simulink model "comp_ctrl"  (R2020b)
settings: Solver=VariableStepAuto  StartTime=0.0  StopTime=2e-3  MaxStep=1e-5  RelTol=1e-3
undefined symbols (not defined in the file or in its folder): den_cos, den_d, L_d, num_cos, num_d, R_s, t_s
libraries: simulink x2
settings Model: PauseTimes=2e-3  Creator=LaptopBN  LastModifiedBy=LaptopBN

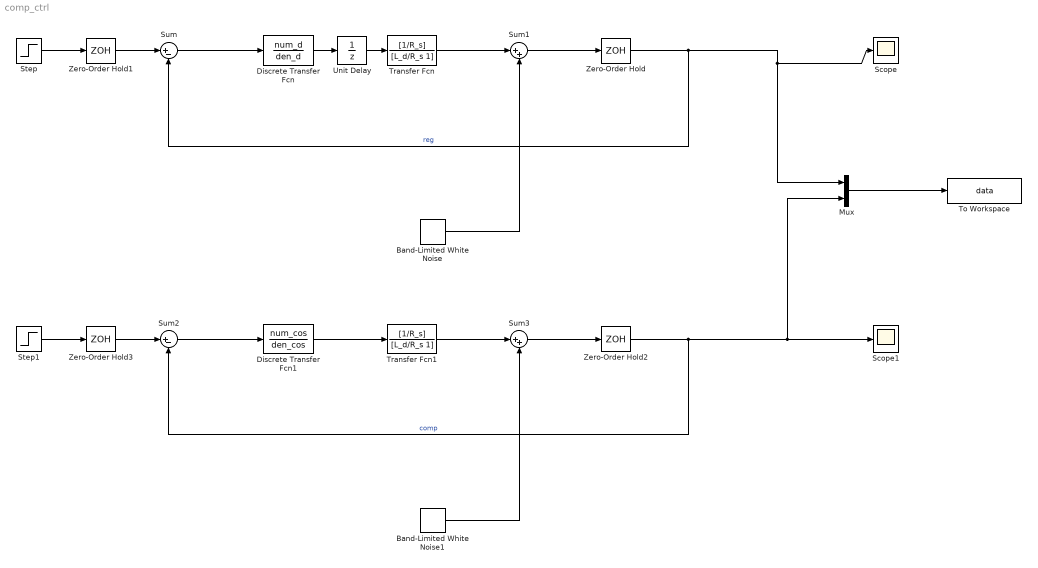
== system comp_ctrl ==
  Band-Limited White Noise : simulink/Sources/Band-Limited White Noise  Cov=[0.002]*t_s  Ts=t_s  seed=[231]
  Band-Limited White Noise1 : simulink/Sources/Band-Limited White Noise  Cov=[0.002]*t_s  Ts=t_s  seed=[232]
  Discrete Transfer Fcn : DiscreteTransferFcn  Numerator=num_d  Denominator=den_d  SampleTime=t_s
  Discrete Transfer Fcn1 : DiscreteTransferFcn  Numerator=num_cos  Denominator=den_cos  SampleTime=t_s
  Mux : Mux  Inputs=2
  Scope : Scope
  Scope1 : Scope
  Step : Step  Time=0  After=10  SampleTime=0
  Step1 : Step  Time=0  After=10  SampleTime=0
  Sum : Sum  Inputs=|+-
  Sum1 : Sum  Inputs=|++
  Sum2 : Sum  Inputs=|+-
  Sum3 : Sum  Inputs=|++
  To Workspace : ToWorkspace  VariableName=data  SaveFormat=Timeseries  SampleTime=-1
  Transfer Fcn : TransferFcn  Numerator=[1/R_s]  Denominator=[L_d/R_s 1]
  Transfer Fcn1 : TransferFcn  Numerator=[1/R_s]  Denominator=[L_d/R_s 1]
  Unit Delay : UnitDelay  SampleTime=-1  HasFrameUpgradeWarning=on
  Zero-Order Hold{,1..3} (4 alike) : ZeroOrderHold  SampleTime=t_s
  wires:
  Discrete Transfer Fcn/1 -> Unit Delay/1
  Sum/1 -> Discrete Transfer Fcn/1
  Step/1 -> Zero-Order Hold1/1
  Transfer Fcn/1 -> Sum1/1
  Sum1/1 -> Zero-Order Hold/1
  Zero-Order Hold/1 -> Sum/2, Mux/1, Scope/1  "reg"
  Zero-Order Hold1/1 -> Sum/1
  Unit Delay/1 -> Transfer Fcn/1
  Band-Limited White Noise/1 -> Sum1/2
  Discrete Transfer Fcn1/1 -> Transfer Fcn1/1
  Band-Limited White Noise1/1 -> Sum3/2
  Zero-Order Hold2/1 -> Sum2/2, Mux/2, Scope1/1  "comp"
  Step1/1 -> Zero-Order Hold3/1
  Zero-Order Hold3/1 -> Sum2/1
  Transfer Fcn1/1 -> Sum3/1
  Sum2/1 -> Discrete Transfer Fcn1/1
  Sum3/1 -> Zero-Order Hold2/1
  Mux/1 -> To Workspace/1
